simulink model "test_ss_mdl"  (Simulink 4.00)
settings: Solver=FixedStepDiscrete  StartTime=0.0  StopTime=120  FixedStep=0.05  RelTol=1e-3
values from neighbouring files (symbols this model uses):
  a = ss_design_ben(Phi_p, Gma_p, C_p, Ts, [5 0.9], [8 0.8])    [test_ss.m]
  controllerData = []    [ControllerDesign_sFcn.m]    (also in controller_redesign.m = newControllerData)
  mdl_p = idss(controllerData.ident.id_mdl)    [test_ss.m]
libraries: cstblocks x2
settings Model: LastModifiedBy=bsaunder

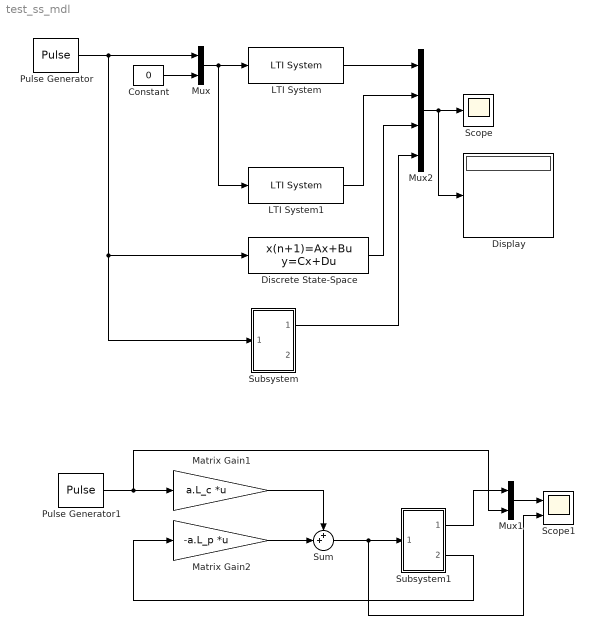
== system test_ss_mdl ==
  Constant : Constant  Value=0
  Discrete State-Space : DiscreteStateSpace  A=mdl_p.A  B=mdl_p.B  C=mdl_p.C  D=0  X0=0  SampleTime=0.05  Realization=auto
      settings: RTWStateStorageClass=Auto
  Display : Display
      settings: Format=short
  LTI System : cstblocks/LTI System  sys=tf(controllerData.ident.id_mdl)  IC=[]
  LTI System1 : cstblocks/LTI System  sys=tf(mdl_p)  IC=[]
  Matrix Gain1 : Gain  Gain=a.L_c  Multiplication=Matrix(K*u)  SaturateOnIntegerOverflow=on
  Matrix Gain2 : Gain  Gain=-a.L_p  Multiplication=Matrix(K*u)  SaturateOnIntegerOverflow=on
  Mux : Mux  Inputs=2
  Mux1 : Mux  Inputs=2
  Mux2 : Mux  Inputs=4
  Pulse Generator : DiscretePulseGenerator  PulseType=Time-based  Amplitude=10  Period=30  PulseWidth=50  PhaseDelay=0  SampleTime=1
  Pulse Generator1 : DiscretePulseGenerator  PulseType=Time-based  Amplitude=10  Period=120  PulseWidth=50  PhaseDelay=0  SampleTime=1
  Scope : Scope
      settings: TimeRange=auto  YMin=-5  YMax=5  SaveToWorkspace=off  SaveName=ScopeData  LimitDataPoints=on  MaxDataPoints=5000
  Scope1 : Scope  NumInputPorts=2
      settings: TimeRange=120  YMin=-2~-5  YMax=12~25  SaveToWorkspace=off  LimitDataPoints=on  MaxDataPoints=5000
  Subsystem : Subsystem
      settings: RTWFcnNameOpts=Auto  RTWFileNameOpts=Auto
  Subsystem1 : Subsystem
      settings: RTWFcnNameOpts=Auto  RTWFileNameOpts=Auto
  Sum : Sum  Inputs=++|  SaturateOnIntegerOverflow=on
  wires:
  Mux/1 -> LTI System/1, LTI System1/1
  Constant/1 -> Mux/2
  Pulse Generator/1 -> Mux/1, Discrete State-Space/1, Subsystem/1(u(k))
  LTI System1/1 -> Mux2/2
  LTI System/1 -> Mux2/1
  Mux2/1 -> Scope/1, Display/1
  Discrete State-Space/1 -> Mux2/3
  Subsystem/1(y(k)) -> Mux2/4
  Pulse Generator1/1 -> Matrix Gain1/1, Mux1/2
  Matrix Gain1/1 -> Sum/1
  Subsystem1/2(x(k)) -> Matrix Gain2/1
  Matrix Gain2/1 -> Sum/2
  Sum/1 -> Subsystem1/1(u(k)), Scope1/2
  Subsystem1/1(y(k)) -> Mux1/1
  Mux1/1 -> Scope1/1

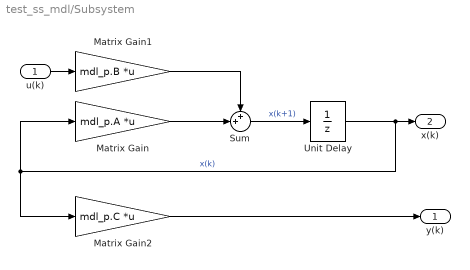
== system test_ss_mdl/Subsystem ==
  u(k) : Inport  Port=1  LatchInput=off
  Matrix Gain : Gain  Gain=mdl_p.A  Multiplication=Matrix(K*u)  SaturateOnIntegerOverflow=on
  Matrix Gain1 : Gain  Gain=mdl_p.B  Multiplication=Matrix(K*u)  SaturateOnIntegerOverflow=on
  Matrix Gain2 : Gain  Gain=mdl_p.C  Multiplication=Matrix(K*u)  SaturateOnIntegerOverflow=on
  Sum : Sum  Inputs=++|  SaturateOnIntegerOverflow=on
  Unit Delay : UnitDelay  X0=0  SampleTime=0.05
      settings: RTWStateStorageClass=Auto
  y(k) : Outport  Port=1
  x(k) : Outport  Port=2
  wires:
  Matrix Gain/1 -> Sum/2
  Matrix Gain1/1 -> Sum/1
  Sum/1 -> Unit Delay/1  "x(k+1)"
  Unit Delay/1 -> Matrix Gain/1, Matrix Gain2/1, x(k)/1  "x(k)"
  u(k)/1 -> Matrix Gain1/1
  Matrix Gain2/1 -> y(k)/1

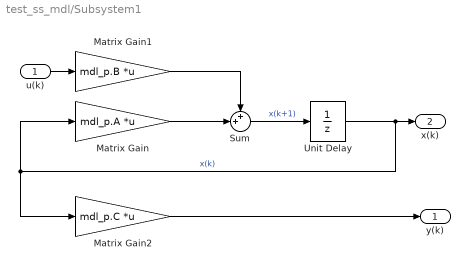
== system test_ss_mdl/Subsystem1 ==
  u(k) : Inport  Port=1  LatchInput=off
  Matrix Gain : Gain  Gain=mdl_p.A  Multiplication=Matrix(K*u)  SaturateOnIntegerOverflow=on
  Matrix Gain1 : Gain  Gain=mdl_p.B  Multiplication=Matrix(K*u)  SaturateOnIntegerOverflow=on
  Matrix Gain2 : Gain  Gain=mdl_p.C  Multiplication=Matrix(K*u)  SaturateOnIntegerOverflow=on
  Sum : Sum  Inputs=++|  SaturateOnIntegerOverflow=on
  Unit Delay : UnitDelay  X0=0  SampleTime=0.05
      settings: RTWStateStorageClass=Auto
  y(k) : Outport  Port=1
  x(k) : Outport  Port=2
  wires:
  Matrix Gain2/1 -> y(k)/1
  u(k)/1 -> Matrix Gain1/1
  Unit Delay/1 -> x(k)/1, Matrix Gain2/1, Matrix Gain/1  "x(k)"
  Sum/1 -> Unit Delay/1  "x(k+1)"
  Matrix Gain1/1 -> Sum/1
  Matrix Gain/1 -> Sum/2
